simulink model "td4"  (R2024a)
settings: Solver=VariableStepAuto  StartTime=0.0  StopTime=10  RelTol=1e-3
libraries: slpidlib x4, dspstat3 x2
settings Model: Creator=tr_nguye  LastModifiedBy=tr_nguye

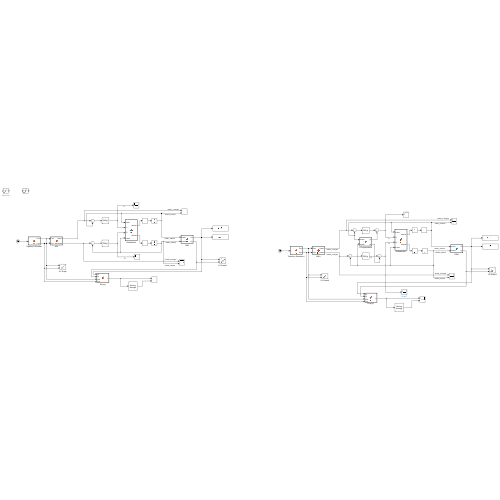
[thumbnail: Simulink's stored preview of the top-level diagram]
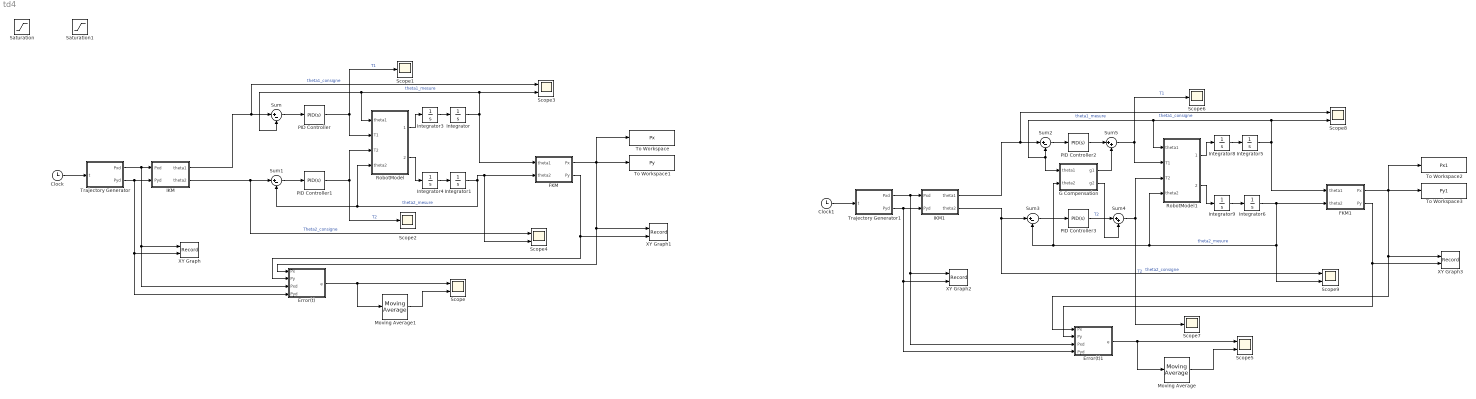
== system td4 ==
  Clock : Clock
      settings: Decimation=1000
  Clock1 : Clock
      settings: Decimation=1000
  Error(t) : MATLAB Function  TreatAsAtomicUnit=on
  Error(t)1 : MATLAB Function  TreatAsAtomicUnit=on
  FKM : MATLAB Function  TreatAsAtomicUnit=on
  FKM1 : MATLAB Function  TreatAsAtomicUnit=on
  G Compensation : MATLAB Function  TreatAsAtomicUnit=on
  IKM : MATLAB Function  TreatAsAtomicUnit=on
  IKM1 : MATLAB Function  TreatAsAtomicUnit=on
  Integrator : Integrator  InitialCondition=-1.2683
  Integrator1 : Integrator  InitialCondition=0.4759
  Integrator{3..4,8..9} (4 alike) : Integrator
  Integrator5 : Integrator  InitialCondition=-1.2683
  Integrator6 : Integrator  InitialCondition=0.4759
  Moving Average : dspstat3/Moving Average  Method=Sliding window  ForgettingFactorPort=off  SpecifyWindowLength=off  WindowLength=4  OverlapLength=3  AllowArbitraryInputLength=off  ForgettingFactor=0.9  SimulateUsing=Interpreted execution
  Moving Average1 : dspstat3/Moving Average  Method=Sliding window  ForgettingFactorPort=off  SpecifyWindowLength=off  WindowLength=4  OverlapLength=3  AllowArbitraryInputLength=off  ForgettingFactor=0.9  SimulateUsing=Interpreted execution
  PID Controller : slpidlib/PID Controller  Controller=PID  Form=Parallel  TimeDomain=Continuous-time  UseExternalTs=off  SampleTime=-1  IntegratorMethod=Forward Euler  FilterMethod=Forward Euler  ControllerParametersSource=internal  P=500  I=500  UseKiTs=off  D=500  UseExternalDerivativeSource=off  N=200  UseFilter=on  TunerSelectOption=Transfer Function Based (PID Tuner App)  InitialConditionSource=internal  InitialConditionForIntegrator=0  InitialConditionForFilter=0  DifferentiatorICPrevScaledInput=0  ExternalReset=none  TrackingMode=off  Kt=1  LimitOutput=off  SatLimitsSource=internal  UpperSaturationLimit=inf  LowerSaturationLimit=-inf  LinearizeAsGain=on  AntiWindupMode=none  Kb=1  LimitIntegrator=off  UpperIntegratorSaturationLimit=inf  LowerIntegratorSaturationLimit=-inf  POutMin=[]  POutMax=[]  IOutMin=[]  IOutMax=[]  DOutMin=[]  DOutMax=[]  NOutMin=[]  NOutMax=[]  SumOutMin=[]  SumOutMax=[]  SaturationOutMin=[]  SaturationOutMax=[]  PParamMin=[]  PParamMax=[]  IParamMin=[]  IParamMax=[]  DParamMin=[]  DParamMax=[]  NParamMin=[]  NParamMax=[]  KbParamMin=[]  KbParamMax=[]  KtParamMin=[]  KtParamMax=[]  KbOutMin=[]  KbOutMax=[]  KtOutMin=[]  KtOutMax=[]  IntegratorOutMin=[]  IntegratorOutMax=[]  FilterOutMin=[]  FilterOutMax=[]  SumI1OutMin=[]  SumI1OutMax=[]  SumI2OutMin=[]  SumI2OutMax=[]  SumI3OutMin=[]  SumI3OutMax=[]  SumI4OutMin=[]  SumI4OutMax=[]  SumDOutMin=[]  SumDOutMax=[]  DifferentiatorOutMin=[]  DifferentiatorOutMax=[]  FilterDiffOutCoefMin=[]  FilterDiffOutCoefMax=[]  ReciprocalOutMin=[]  ReciprocalOutMax=[]  SumDenOutMin=[]  SumDenOutMax=[]  SumNumOutMin=[]  SumNumOutMax=[]  DivideOutMin=[]  DivideOutMax=[]  UdiffTsProdOutMin=[]  UdiffTsProdOutMax=[]  NTsProdOutMin=[]  NTsProdOutMax=[]  UintegralTsProdOutMin=[]  UintegralTsProdOutMax=[]  UngainTsProdOutMin=[]  UngainTsProdOutMax=[]  ClampingZeroOutDataTypeStr=Inherit: Inherit via back propagation  ClampingZeroOutMin=[]  ClampingZeroOutMax=[]  FilterDenConstantOutDataTypeStr=Inherit: Inherit via back propagation  FilterDenConstantOutMin=[]  FilterDenConstantOutMax=[]  PCopyOutDataTypeStr=Inherit: Inherit via back propagation  PCopyOutMin=[]  PCopyOutMax=[]  NCopyOutDataTypeStr=Inherit: Inherit via back propagation  NCopyOutMin=[]  NCopyOutMax=[]  IntegratorContinuousStateAttributes=''  IntegratorStateMustResolveToSignalObject=off  IntegratorRTWStateStorageClass=Auto  FilterContinuousStateAttributes=''  FilterStateMustResolveToSignalObject=off  FilterRTWStateStorageClass=Auto  ParallelPVariant=InternalParameters  IdealPVariant=Disabled  IVariant=InternalParameters  DVariant=InternalParameters  IntegratorVariant=Continuous  SatVariant=Disabled  AWVariant=Passthrough  PCopyVariant=Disabled  TRVariant=Disabled  FdbkBlocksVariant=Forward  IdealPFdbkVariant=Disabled  SatFdbkVariant=Disabled  DerivativeFilterVariant=ContFilter  NVariant=InternalParameters  NCopyVariant=Disabled  FilterICVariant=InternalICsFilter  IntegratorICVariant=InternalICs  ExternalResetVariant=Disabled  TRSumVariant=Passthrough  SumFdbkVariant=Disabled  SumVariant=Sum_PID  TsampFilterVariant=InternalTs  TsampNgainVariant=Passthrough  TsampIntegralVariant=Disabled_SignalSpec  ExternalSaturationOutDataTypeStr=Inherit: Same as second input  DerivativeSourceVariant=ErrorSignal
  PID Controller1 : slpidlib/PID Controller  Controller=PID  Form=Parallel  TimeDomain=Continuous-time  UseExternalTs=off  SampleTime=-1  IntegratorMethod=Forward Euler  FilterMethod=Forward Euler  ControllerParametersSource=internal  P=500  I=300  UseKiTs=off  D=300  UseExternalDerivativeSource=off  N=100  UseFilter=on  TunerSelectOption=Transfer Function Based (PID Tuner App)  InitialConditionSource=internal  InitialConditionForIntegrator=0  InitialConditionForFilter=0  DifferentiatorICPrevScaledInput=0  ExternalReset=none  TrackingMode=off  Kt=1  LimitOutput=off  SatLimitsSource=internal  UpperSaturationLimit=inf  LowerSaturationLimit=-inf  LinearizeAsGain=on  AntiWindupMode=none  Kb=1  LimitIntegrator=off  UpperIntegratorSaturationLimit=inf  LowerIntegratorSaturationLimit=-inf  POutMin=[]  POutMax=[]  IOutMin=[]  IOutMax=[]  DOutMin=[]  DOutMax=[]  NOutMin=[]  NOutMax=[]  SumOutMin=[]  SumOutMax=[]  SaturationOutMin=[]  SaturationOutMax=[]  PParamMin=[]  PParamMax=[]  IParamMin=[]  IParamMax=[]  DParamMin=[]  DParamMax=[]  NParamMin=[]  NParamMax=[]  KbParamMin=[]  KbParamMax=[]  KtParamMin=[]  KtParamMax=[]  KbOutMin=[]  KbOutMax=[]  KtOutMin=[]  KtOutMax=[]  IntegratorOutMin=[]  IntegratorOutMax=[]  FilterOutMin=[]  FilterOutMax=[]  SumI1OutMin=[]  SumI1OutMax=[]  SumI2OutMin=[]  SumI2OutMax=[]  SumI3OutMin=[]  SumI3OutMax=[]  SumI4OutMin=[]  SumI4OutMax=[]  SumDOutMin=[]  SumDOutMax=[]  DifferentiatorOutMin=[]  DifferentiatorOutMax=[]  FilterDiffOutCoefMin=[]  FilterDiffOutCoefMax=[]  ReciprocalOutMin=[]  ReciprocalOutMax=[]  SumDenOutMin=[]  SumDenOutMax=[]  SumNumOutMin=[]  SumNumOutMax=[]  DivideOutMin=[]  DivideOutMax=[]  UdiffTsProdOutMin=[]  UdiffTsProdOutMax=[]  NTsProdOutMin=[]  NTsProdOutMax=[]  UintegralTsProdOutMin=[]  UintegralTsProdOutMax=[]  UngainTsProdOutMin=[]  UngainTsProdOutMax=[]  ClampingZeroOutDataTypeStr=Inherit: Inherit via back propagation  ClampingZeroOutMin=[]  ClampingZeroOutMax=[]  FilterDenConstantOutDataTypeStr=Inherit: Inherit via back propagation  FilterDenConstantOutMin=[]  FilterDenConstantOutMax=[]  PCopyOutDataTypeStr=Inherit: Inherit via back propagation  PCopyOutMin=[]  PCopyOutMax=[]  NCopyOutDataTypeStr=Inherit: Inherit via back propagation  NCopyOutMin=[]  NCopyOutMax=[]  IntegratorContinuousStateAttributes=''  IntegratorStateMustResolveToSignalObject=off  IntegratorRTWStateStorageClass=Auto  FilterContinuousStateAttributes=''  FilterStateMustResolveToSignalObject=off  FilterRTWStateStorageClass=Auto  ParallelPVariant=InternalParameters  IdealPVariant=Disabled  IVariant=InternalParameters  DVariant=InternalParameters  IntegratorVariant=Continuous  SatVariant=Disabled  AWVariant=Passthrough  PCopyVariant=Disabled  TRVariant=Disabled  FdbkBlocksVariant=Forward  IdealPFdbkVariant=Disabled  SatFdbkVariant=Disabled  DerivativeFilterVariant=ContFilter  NVariant=InternalParameters  NCopyVariant=Disabled  FilterICVariant=InternalICsFilter  IntegratorICVariant=InternalICs  ExternalResetVariant=Disabled  TRSumVariant=Passthrough  SumFdbkVariant=Disabled  SumVariant=Sum_PID  TsampFilterVariant=InternalTs  TsampNgainVariant=Passthrough  TsampIntegralVariant=Disabled_SignalSpec  ExternalSaturationOutDataTypeStr=Inherit: Same as second input  DerivativeSourceVariant=ErrorSignal
  PID Controller2 : slpidlib/PID Controller  Controller=PID  Form=Parallel  TimeDomain=Continuous-time  UseExternalTs=off  SampleTime=-1  IntegratorMethod=Forward Euler  FilterMethod=Forward Euler  ControllerParametersSource=internal  P=500  I=500  UseKiTs=off  D=500  UseExternalDerivativeSource=off  N=200  UseFilter=on  TunerSelectOption=Transfer Function Based (PID Tuner App)  InitialConditionSource=internal  InitialConditionForIntegrator=0  InitialConditionForFilter=0  DifferentiatorICPrevScaledInput=0  ExternalReset=none  TrackingMode=off  Kt=1  LimitOutput=off  SatLimitsSource=internal  UpperSaturationLimit=inf  LowerSaturationLimit=-inf  LinearizeAsGain=on  AntiWindupMode=none  Kb=1  LimitIntegrator=off  UpperIntegratorSaturationLimit=inf  LowerIntegratorSaturationLimit=-inf  POutMin=[]  POutMax=[]  IOutMin=[]  IOutMax=[]  DOutMin=[]  DOutMax=[]  NOutMin=[]  NOutMax=[]  SumOutMin=[]  SumOutMax=[]  SaturationOutMin=[]  SaturationOutMax=[]  PParamMin=[]  PParamMax=[]  IParamMin=[]  IParamMax=[]  DParamMin=[]  DParamMax=[]  NParamMin=[]  NParamMax=[]  KbParamMin=[]  KbParamMax=[]  KtParamMin=[]  KtParamMax=[]  KbOutMin=[]  KbOutMax=[]  KtOutMin=[]  KtOutMax=[]  IntegratorOutMin=[]  IntegratorOutMax=[]  FilterOutMin=[]  FilterOutMax=[]  SumI1OutMin=[]  SumI1OutMax=[]  SumI2OutMin=[]  SumI2OutMax=[]  SumI3OutMin=[]  SumI3OutMax=[]  SumI4OutMin=[]  SumI4OutMax=[]  SumDOutMin=[]  SumDOutMax=[]  DifferentiatorOutMin=[]  DifferentiatorOutMax=[]  FilterDiffOutCoefMin=[]  FilterDiffOutCoefMax=[]  ReciprocalOutMin=[]  ReciprocalOutMax=[]  SumDenOutMin=[]  SumDenOutMax=[]  SumNumOutMin=[]  SumNumOutMax=[]  DivideOutMin=[]  DivideOutMax=[]  UdiffTsProdOutMin=[]  UdiffTsProdOutMax=[]  NTsProdOutMin=[]  NTsProdOutMax=[]  UintegralTsProdOutMin=[]  UintegralTsProdOutMax=[]  UngainTsProdOutMin=[]  UngainTsProdOutMax=[]  ClampingZeroOutDataTypeStr=Inherit: Inherit via back propagation  ClampingZeroOutMin=[]  ClampingZeroOutMax=[]  FilterDenConstantOutDataTypeStr=Inherit: Inherit via back propagation  FilterDenConstantOutMin=[]  FilterDenConstantOutMax=[]  PCopyOutDataTypeStr=Inherit: Inherit via back propagation  PCopyOutMin=[]  PCopyOutMax=[]  NCopyOutDataTypeStr=Inherit: Inherit via back propagation  NCopyOutMin=[]  NCopyOutMax=[]  IntegratorContinuousStateAttributes=''  IntegratorStateMustResolveToSignalObject=off  IntegratorRTWStateStorageClass=Auto  FilterContinuousStateAttributes=''  FilterStateMustResolveToSignalObject=off  FilterRTWStateStorageClass=Auto  ParallelPVariant=InternalParameters  IdealPVariant=Disabled  IVariant=InternalParameters  DVariant=InternalParameters  IntegratorVariant=Continuous  SatVariant=Disabled  AWVariant=Passthrough  PCopyVariant=Disabled  TRVariant=Disabled  FdbkBlocksVariant=Forward  IdealPFdbkVariant=Disabled  SatFdbkVariant=Disabled  DerivativeFilterVariant=ContFilter  NVariant=InternalParameters  NCopyVariant=Disabled  FilterICVariant=InternalICsFilter  IntegratorICVariant=InternalICs  ExternalResetVariant=Disabled  TRSumVariant=Passthrough  SumFdbkVariant=Disabled  SumVariant=Sum_PID  TsampFilterVariant=InternalTs  TsampNgainVariant=Passthrough  TsampIntegralVariant=Disabled_SignalSpec  ExternalSaturationOutDataTypeStr=Inherit: Same as second input  DerivativeSourceVariant=ErrorSignal
  PID Controller3 : slpidlib/PID Controller  Controller=PID  Form=Parallel  TimeDomain=Continuous-time  UseExternalTs=off  SampleTime=-1  IntegratorMethod=Forward Euler  FilterMethod=Forward Euler  ControllerParametersSource=internal  P=500  I=500  UseKiTs=off  D=500  UseExternalDerivativeSource=off  N=100  UseFilter=on  TunerSelectOption=Transfer Function Based (PID Tuner App)  InitialConditionSource=internal  InitialConditionForIntegrator=0  InitialConditionForFilter=0  DifferentiatorICPrevScaledInput=0  ExternalReset=none  TrackingMode=off  Kt=1  LimitOutput=off  SatLimitsSource=internal  UpperSaturationLimit=inf  LowerSaturationLimit=-inf  LinearizeAsGain=on  AntiWindupMode=none  Kb=1  LimitIntegrator=off  UpperIntegratorSaturationLimit=inf  LowerIntegratorSaturationLimit=-inf  POutMin=[]  POutMax=[]  IOutMin=[]  IOutMax=[]  DOutMin=[]  DOutMax=[]  NOutMin=[]  NOutMax=[]  SumOutMin=[]  SumOutMax=[]  SaturationOutMin=[]  SaturationOutMax=[]  PParamMin=[]  PParamMax=[]  IParamMin=[]  IParamMax=[]  DParamMin=[]  DParamMax=[]  NParamMin=[]  NParamMax=[]  KbParamMin=[]  KbParamMax=[]  KtParamMin=[]  KtParamMax=[]  KbOutMin=[]  KbOutMax=[]  KtOutMin=[]  KtOutMax=[]  IntegratorOutMin=[]  IntegratorOutMax=[]  FilterOutMin=[]  FilterOutMax=[]  SumI1OutMin=[]  SumI1OutMax=[]  SumI2OutMin=[]  SumI2OutMax=[]  SumI3OutMin=[]  SumI3OutMax=[]  SumI4OutMin=[]  SumI4OutMax=[]  SumDOutMin=[]  SumDOutMax=[]  DifferentiatorOutMin=[]  DifferentiatorOutMax=[]  FilterDiffOutCoefMin=[]  FilterDiffOutCoefMax=[]  ReciprocalOutMin=[]  ReciprocalOutMax=[]  SumDenOutMin=[]  SumDenOutMax=[]  SumNumOutMin=[]  SumNumOutMax=[]  DivideOutMin=[]  DivideOutMax=[]  UdiffTsProdOutMin=[]  UdiffTsProdOutMax=[]  NTsProdOutMin=[]  NTsProdOutMax=[]  UintegralTsProdOutMin=[]  UintegralTsProdOutMax=[]  UngainTsProdOutMin=[]  UngainTsProdOutMax=[]  ClampingZeroOutDataTypeStr=Inherit: Inherit via back propagation  ClampingZeroOutMin=[]  ClampingZeroOutMax=[]  FilterDenConstantOutDataTypeStr=Inherit: Inherit via back propagation  FilterDenConstantOutMin=[]  FilterDenConstantOutMax=[]  PCopyOutDataTypeStr=Inherit: Inherit via back propagation  PCopyOutMin=[]  PCopyOutMax=[]  NCopyOutDataTypeStr=Inherit: Inherit via back propagation  NCopyOutMin=[]  NCopyOutMax=[]  IntegratorContinuousStateAttributes=''  IntegratorStateMustResolveToSignalObject=off  IntegratorRTWStateStorageClass=Auto  FilterContinuousStateAttributes=''  FilterStateMustResolveToSignalObject=off  FilterRTWStateStorageClass=Auto  ParallelPVariant=InternalParameters  IdealPVariant=Disabled  IVariant=InternalParameters  DVariant=InternalParameters  IntegratorVariant=Continuous  SatVariant=Disabled  AWVariant=Passthrough  PCopyVariant=Disabled  TRVariant=Disabled  FdbkBlocksVariant=Forward  IdealPFdbkVariant=Disabled  SatFdbkVariant=Disabled  DerivativeFilterVariant=ContFilter  NVariant=InternalParameters  NCopyVariant=Disabled  FilterICVariant=InternalICsFilter  IntegratorICVariant=InternalICs  ExternalResetVariant=Disabled  TRSumVariant=Passthrough  SumFdbkVariant=Disabled  SumVariant=Sum_PID  TsampFilterVariant=InternalTs  TsampNgainVariant=Passthrough  TsampIntegralVariant=Disabled_SignalSpec  ExternalSaturationOutDataTypeStr=Inherit: Same as second input  DerivativeSourceVariant=ErrorSignal
  RobotModel : MATLAB Function  TreatAsAtomicUnit=on
  RobotModel1 : MATLAB Function  TreatAsAtomicUnit=on
  Saturation : Saturate  UpperLimit=24  LowerLimit=-24
  Saturation1 : Saturate  UpperLimit=24  LowerLimit=-24
  Scope{,3..5,8..9} (6 alike) : Scope  NumInputPorts=2
  Scope{1..2,6..7} (4 alike) : Scope
  Sum{,1..3} (4 alike) : Sum  Inputs=|+-
  Sum4 : Sum  Inputs=|++
  Sum5 : Sum  Inputs=|++
  To Workspace : ToWorkspace  VariableName=Px  SaveFormat=Timeseries  SampleTime=-1
  To Workspace1 : ToWorkspace  VariableName=Py  SaveFormat=Timeseries  SampleTime=-1
  To Workspace2 : ToWorkspace  VariableName=Px1  SaveFormat=Timeseries  SampleTime=-1
  To Workspace3 : ToWorkspace  VariableName=Py1  SaveFormat=Timeseries  SampleTime=-1
  Trajectory Generator : MATLAB Function  TreatAsAtomicUnit=on
  Trajectory Generator1 : MATLAB Function  TreatAsAtomicUnit=on
  XY Graph : Record  FileSettingsInternal="{\"entries\":[{\"content\":{\"excelSettings\":{\"content\":{},\"type\":\"Streamout.ExcelSettings\"}},\"type\":\"Streamout.FileSettingStorage\",\"uuid\":\"\"}],\"packageUris\":[\"http:\\/\\/schema.mathworks.com\\/mf0\\/streamout_blocks\\/R2020a\"],\"version\":\"1.0\"}"  Layout=[1 1]  SignalsInternal="{\"entries\":[{\"content\":{\"signals\":[{\"content\":{\"blockPath\":[],\"dimensions\":[1],\"domain\":\"\",\"lineColor\":\"#a2142f\",\"plots\":[ 1 ],\"port\":1,\"sid\":[\"\"],\"signalID\":1,\"signalName\":\"Trajectory Generator:1\"},\"type\":\"RecordBlkView.Signal\",\"uuid\":\"\"},{\"content\":{\"blockPath\":[],\"dimensions\":[1],\"domain\":\"\",\"lineColor\":\"#139fff\",\"plots\":[ 1 ],\"port\":2,\"sid\":[\"\"],\"signalID\":2,\"signalName\":\"Trajectory Generator:2\"},\"type\":\"RecordBlkView.Signal\",\"uuid\":\"\"}]},\"type\":\"RecordBlkView.InputSignals\",\"uuid\":\"\"}],\"packageUris\":[\"http:\\/\\/schema.mathworks.com\\/mf0\\/streamout_blocks\\/R2020a\"],\"version\":\"1.0\"}"  VisualizationBindings="{\"xyplotplugin\":{\"info\":[{\"series\":[{\"bindingParametersList\":[{\"parameter\":\"X-Axis\",\"signalID\":1,\"signalName\":\"Trajectory Generator:1\"},{\"parameter\":\"Y-Axis\",\"signalID\":2,\"signalName\":\"Trajectory Generator:2\"}],\"seriesID\":0}],\"subplotID\":1}]}}"  CompatibilityTag=XY
  XY Graph1 : Record  FileSettingsInternal="{\"entries\":[{\"content\":{\"excelSettings\":{\"content\":{},\"type\":\"Streamout.ExcelSettings\"}},\"type\":\"Streamout.FileSettingStorage\",\"uuid\":\"\"}],\"packageUris\":[\"http:\\/\\/schema.mathworks.com\\/mf0\\/streamout_blocks\\/R2020a\"],\"version\":\"1.0\"}"  Layout=[1 1]  SignalsInternal="{\"entries\":[{\"content\":{\"signals\":[{\"content\":{\"blockPath\":[],\"dimensions\":[1],\"domain\":\"\",\"lineColor\":\"#a2142f\",\"plots\":[ 1 ],\"port\":1,\"sid\":[\"\"],\"signalID\":1,\"signalName\":\"FKM:1\"},\"type\":\"RecordBlkView.Signal\",\"uuid\":\"\"},{\"content\":{\"blockPath\":[],\"dimensions\":[1],\"domain\":\"\",\"lineColor\":\"#139fff\",\"plots\":[ 1 ],\"port\":2,\"sid\":[\"\"],\"signalID\":2,\"signalName\":\"FKM:2\"},\"type\":\"RecordBlkView.Signal\",\"uuid\":\"\"}]},\"type\":\"RecordBlkView.InputSignals\",\"uuid\":\"\"}],\"packageUris\":[\"http:\\/\\/schema.mathworks.com\\/mf0\\/streamout_blocks\\/R2020a\"],\"version\":\"1.0\"}"  VisualizationBindings="{\"xyplotplugin\":{\"info\":[{\"series\":[{\"bindingParametersList\":[{\"parameter\":\"X-Axis\",\"signalID\":1,\"signalName\":\"FKM:1\"},{\"parameter\":\"Y-Axis\",\"signalID\":2,\"signalName\":\"FKM:2\"}],\"seriesID\":0}],\"subplotID\":1}]}}"  CompatibilityTag=XY
  XY Graph2 : Record  FileSettingsInternal="{\"entries\":[{\"content\":{\"excelSettings\":{\"content\":{},\"type\":\"Streamout.ExcelSettings\"}},\"type\":\"Streamout.FileSettingStorage\",\"uuid\":\"\"}],\"packageUris\":[\"http:\\/\\/schema.mathworks.com\\/mf0\\/streamout_blocks\\/R2020a\"],\"version\":\"1.0\"}"  Layout=[1 1]  SignalsInternal="{\"entries\":[{\"content\":{\"signals\":[{\"content\":{\"blockPath\":[],\"dimensions\":[1],\"domain\":\"\",\"lineColor\":\"#a2142f\",\"plots\":[ 1 ],\"port\":1,\"sid\":[\"\"],\"signalID\":1,\"signalName\":\"Trajectory Generator1:1\"},\"type\":\"RecordBlkView.Signal\",\"uuid\":\"\"},{\"content\":{\"blockPath\":[],\"dimensions\":[1],\"domain\":\"\",\"lineColor\":\"#139fff\",\"plots\":[ 1 ],\"port\":2,\"sid\":[\"\"],\"signalID\":2,\"signalName\":\"Trajectory Generator1:2\"},\"type\":\"RecordBlkView.Signal\",\"uuid\":\"\"}]},\"type\":\"RecordBlkView.InputSignals\",\"uuid\":\"\"}],\"packageUris\":[\"http:\\/\\/schema.mathworks.com\\/mf0\\/streamout_blocks\\/R2020a\"],\"version\":\"1.0\"}"  VisualizationBindings="{\"xyplotplugin\":{\"info\":[{\"series\":[{\"bindingParametersList\":[{\"parameter\":\"X-Axis\",\"signalID\":1,\"signalName\":\"Trajectory Generator1:1\"},{\"parameter\":\"Y-Axis\",\"signalID\":2,\"signalName\":\"Trajectory Generator1:2\"}],\"seriesID\":0}],\"subplotID\":1}]}}"  CompatibilityTag=XY
  XY Graph3 : Record  FileSettingsInternal="{\"entries\":[{\"content\":{\"excelSettings\":{\"content\":{},\"type\":\"Streamout.ExcelSettings\"}},\"type\":\"Streamout.FileSettingStorage\",\"uuid\":\"\"}],\"packageUris\":[\"http:\\/\\/schema.mathworks.com\\/mf0\\/streamout_blocks\\/R2020a\"],\"version\":\"1.0\"}"  Layout=[1 1]  SignalsInternal="{\"entries\":[{\"content\":{\"signals\":[{\"content\":{\"blockPath\":[],\"dimensions\":[1],\"domain\":\"\",\"lineColor\":\"#a2142f\",\"plots\":[ 1 ],\"port\":1,\"sid\":[\"\"],\"signalID\":1,\"signalName\":\"FKM1:1\"},\"type\":\"RecordBlkView.Signal\",\"uuid\":\"\"},{\"content\":{\"blockPath\":[],\"dimensions\":[1],\"domain\":\"\",\"lineColor\":\"#139fff\",\"plots\":[ 1 ],\"port\":2,\"sid\":[\"\"],\"signalID\":2,\"signalName\":\"FKM1:2\"},\"type\":\"RecordBlkView.Signal\",\"uuid\":\"\"}]},\"type\":\"RecordBlkView.InputSignals\",\"uuid\":\"\"}],\"packageUris\":[\"http:\\/\\/schema.mathworks.com\\/mf0\\/streamout_blocks\\/R2020a\"],\"version\":\"1.0\"}"  VisualizationBindings="{\"xyplotplugin\":{\"info\":[{\"series\":[{\"bindingParametersList\":[{\"parameter\":\"X-Axis\",\"signalID\":1,\"signalName\":\"FKM1:1\"},{\"parameter\":\"Y-Axis\",\"signalID\":2,\"signalName\":\"FKM1:2\"}],\"seriesID\":0}],\"subplotID\":1}]}}"  CompatibilityTag=XY
  wires:
  FKM/2(Py) -> Error(t)/2(Py), XY Graph1/2
  Moving Average1/1 -> Scope/2
  Error(t)/1(e) -> Moving Average1/1, Scope/1
  FKM/1(Px) -> Error(t)/1(Px), XY Graph1/1, To Workspace1/1, To Workspace/1
  PID Controller1/1 -> RobotModel/3(T2), Scope2/1  "T2"
  Sum1/1 -> PID Controller1/1
  Sum/1 -> PID Controller/1
  Trajectory Generator/1(Pxd) -> Error(t)/3(Pxd), XY Graph/1, IKM/1(Pxd)
  Clock/1 -> Trajectory Generator/1(t)
  Integrator/1 -> Sum/2, RobotModel/1(theta1), Scope3/2, FKM/1(theta1)  "theta1_mesure"
  Integrator1/1 -> RobotModel/4(theta2), Sum1/2, FKM/2(theta2), Scope4/2  "theta2_mesure"
  PID Controller/1 -> RobotModel/2(T1), Scope1/1  "T1"
  Trajectory Generator/2(Pyd) -> Error(t)/4(Pyd), XY Graph/2, IKM/2(Pyd)
  IKM/2(theta2) -> Scope4/1, Sum1/1  "Theta2_consigne"
  IKM/1(theta1) -> Sum/1, Scope3/1  "theta1_consigne"
  Integrator3/1 -> Integrator/1
  RobotModel/1(atheta1) -> Integrator3/1
  Integrator4/1 -> Integrator1/1
  RobotModel/2(atheta2) -> Integrator4/1
  Integrator9/1 -> Integrator6/1
  RobotModel1/2(atheta2) -> Integrator9/1
  IKM1/2(theta2) -> Sum3/1, Scope9/1  "theta2_consigne"
  IKM1/1(theta1) -> Sum2/1, Scope8/1  "theta1_consigne"
  Trajectory Generator1/1(Pxd) -> Error(t)1/3(Pxd), XY Graph2/1, IKM1/1(Pxd)
  RobotModel1/1(atheta1) -> Integrator8/1
  Trajectory Generator1/2(Pyd) -> XY Graph2/2, Error(t)1/4(Pyd), IKM1/2(Pyd)
  Integrator6/1 -> FKM1/2(theta2), RobotModel1/4(theta2), G Compensation/2(theta2), Sum3/2, Scope9/2  "theta2_mesure"
  Integrator5/1 -> G Compensation/1(theta1), Sum2/2, RobotModel1/1(theta1), Scope8/2, FKM1/1(theta1)  "theta1_mesure"
  Error(t)1/1(e) -> Moving Average/1, Scope5/1
  Integrator8/1 -> Integrator5/1
  FKM1/1(Px) -> Error(t)1/1(Px), XY Graph3/1, To Workspace3/1, To Workspace2/1
  FKM1/2(Py) -> Error(t)1/2(Py), XY Graph3/2
  Sum3/1 -> PID Controller3/1
  Sum2/1 -> PID Controller2/1
  Clock1/1 -> Trajectory Generator1/1(t)
  PID Controller2/1 -> Sum5/1
  Sum5/1 -> Scope6/1, RobotModel1/2(T1)  "T1"
  PID Controller3/1 -> Sum4/1  "T2"
  Sum4/1 -> RobotModel1/3(T2), Scope7/1  "T2"
  G Compensation/1(g1) -> Sum5/2
  Moving Average/1 -> Scope5/2
  G Compensation/2(g2) -> Sum4/2

== matlab function td4/Trajectory Generator1 ==
  data: t input; Pxd output; Pyd output
function [Pxd, Pyd]= fcn(t)
V = 0.5;
A =  2;
tau = V/A;

x_0 = -0.5;
x_1 = 0.5;

T = abs(x_1 - x_0)/V - tau;

Pxd = 0.3;
Pyd = x_0;
if (t >= 0) && (t <= tau)
    Pyd = 1/2 * A * t^2 +x_0;
elseif (t >= tau) && (t <= tau+ T)
    Pyd = V * (t - tau/2) + x_0;
elseif (t >= T + tau) && (t <= T + 2*tau)
    Pyd = -(1/2)*A*(t-2*tau-T)^2+x_1;
else
    Pyd = x_1;
end

== matlab function td4/G Compensation ==
  data: theta1 input; g1 output; theta2 input; g2 output
function [g1, g2] = fcn(theta1, theta2)
l1 = 0.3;
l2 = 0.3;
m1 = 1;
m2 = 1;
g = 9.806;
g1 = m2*l2*cos(theta1 + theta2) + (m1 + m2)*l1*g*cos(theta1);
g2 = m2*l2*cos(theta1 + theta2);

== matlab function td4/Trajectory Generator ==
  data: t input; Pxd output; Pyd output
function [Pxd, Pyd]= fcn(t)
V = 0.5;
A =  2;
tau = V/A;

x_0 = -0.5;
x_1 = 0.5;

T = abs(x_1 - x_0)/V - tau;

Pxd = 0.3;
Pyd = x_0;
if (t >= 0) && (t <= tau)
    Pyd = 1/2 * A * t^2 +x_0;
elseif (t >= tau) && (t <= tau+ T)
    Pyd = V * (t - tau/2) + x_0;
elseif (t >= T + tau) && (t <= T + 2*tau)
    Pyd = -(1/2)*A*(t-2*tau-T)^2+x_1;
else
    Pyd = x_1;
end

== matlab function td4/IKM ==
  data: Pxd input; theta1 output; Pyd input; theta2 output
function [theta1, theta2]= fcn(Pxd,Pyd)
l_1 = 0.3;
l_2 = 0.3;
theta1 = 0;
theta2 = 0;

theta2 = acos((Pxd^2 + Pyd^2 - l_1^2 - l_2^2)/(2*l_1*l_2));
theta1 = atan2(-l_2*sin(theta2)*Pxd + (l_1 + l_2*cos(theta2))*Pyd, l_2*sin(theta2)*Pyd + (l_1 +l_2*cos(theta2))*Pxd);

== matlab function td4/FKM ==
  data: theta1 input; Px output; Py output; theta2 input
function [Px, Py] = fcn(theta1, theta2)
l_1 = 0.3;
l_2 = 0.3;
Px = l_1*cos(theta1) + l_2*cos(theta1 + theta2);
Py = l_1*sin(theta1) + l_2*sin(theta1 + theta2);

== matlab function td4/Error(t) ==
  data: Px input; Py input; Pxd input; e output; Pyd input
function e= fcn(Px, Py, Pxd, Pyd)
    e = sqrt((Pxd-Px)^2+(Pyd-Py)^2);
    
    % fun = @e;
    % tau = 0.25;
    % T = 1.75;
    % t_final = 2*tau+T;
    % e_total = integral(@e,0,t_final);
end

== matlab function td4/RobotModel ==
  data: theta1 input; T1 input; atheta1 output; atheta2 output; T2 input; theta2 input
function [atheta1, atheta2]= fcn(theta1, T1, T2, theta2)
l1 = 0.5;
l2 = 0.5;
m1 = 1;
m2 = 1;
g = 9.81;

M11 = m2*l2^2 + (m1+m2)*(l1^2)+2*l1*l2*m2*cos(theta2);
M12 = m2*l2^2 + l1*l2*m2*cos(theta2);
M21 = m2*l2^2 + l1*l2*m2*cos(theta2);
M22 = m2*l2^2;
M = [M11 M12
     M21 M22];
G11 = m2*l2*g*cos(theta1+theta2) + (m1+m2)*l1*g*cos(theta1);
G21 = m2*l2*g*cos(theta1 + theta2);
G = [G11
     G21];

T = [T1
     T2];

atheta = M\(T-G);
atheta1 = atheta(1);
atheta2 = atheta(2);
end

== matlab function td4/Error(t)1 ==
  data: Px input; Py input; Pxd input; e output; Pyd input
function e= fcn(Px, Py, Pxd, Pyd)
    e = sqrt((Pxd-Px)^2+(Pyd-Py)^2);
    
    % fun = @e;
    % tau = 0.25;
    % T = 1.75;
    % t_final = 2*tau+T;
    % e_total = integral(@e,0,t_final);
end

== matlab function td4/FKM1 ==
  data: theta1 input; Px output; Py output; theta2 input
function [Px, Py] = fcn(theta1, theta2)
l_1 = 0.3;
l_2 = 0.3;
Px = l_1*cos(theta1) + l_2*cos(theta1 + theta2);
Py = l_1*sin(theta1) + l_2*sin(theta1 + theta2);

== matlab function td4/IKM1 ==
  data: Pxd input; theta1 output; Pyd input; theta2 output
function [theta1, theta2]= fcn(Pxd,Pyd)
l_1 = 0.3;
l_2 = 0.3;
theta1 = 0;
theta2 = 0;

theta2 = acos((Pxd^2 + Pyd^2 - l_1^2 - l_2^2)/(2*l_1*l_2));
theta1 = atan2(-l_2*sin(theta2)*Pxd + (l_1 + l_2*cos(theta2))*Pyd, l_2*sin(theta2)*Pyd + (l_1 +l_2*cos(theta2))*Pxd);

== matlab function td4/RobotModel1 ==
  data: theta1 input; T1 input; atheta1 output; atheta2 output; T2 input; theta2 input
function [atheta1, atheta2]= fcn(theta1, T1, T2, theta2)
l1 = 0.5;
l2 = 0.5;
m1 = 1;
m2 = 1;
g = 9.81;

M11 = m2*l2^2 + (m1+m2)*(l1^2)+2*l1*l2*m2*cos(theta2);
M12 = m2*l2^2 + l1*l2*m2*cos(theta2);
M21 = m2*l2^2 + l1*l2*m2*cos(theta2);
M22 = m2*l2^2;
M = [M11 M12
     M21 M22];
G11 = m2*l2*g*cos(theta1+theta2) + (m1+m2)*l1*g*cos(theta1);
G21 = m2*l2*g*cos(theta1 + theta2);
G = [G11
     G21];

T = [T1
     T2];

atheta = M\(T-G);
atheta1 = atheta(1);
atheta2 = atheta(2);
end
